simulink model "wavelet_transform_int"  (R2024b)
settings: Solver=FixedStepDiscrete  StartTime=0.0  StopTime=10.0  RelTol=1e-3
InitFcn:
  | n=50;
  | 
  | fprintf('Size of matrix A: n = %d\n', n);
libraries: simulink x1
settings Model: DataTypeOverride=Off  Creator=valen  LastModifiedBy=valen
settings SolverCC: AlgebraicLoopSolver=TrustRegion
settings DataIOCC: LimitDataPoints=on  SaveOutput=off  SaveTime=off
settings OptimizationCC: BlockReduction=off  ConditionallyExecuteInputs=off  DefaultParameterBehavior=Inlined  LifeSpan=inf
settings DebuggingCC: AlgebraicLoopMsg=error  SingleTaskRateTransMsg=error  UnconnectedInputMsg=warning  UnconnectedOutputMsg=warning  UnconnectedLineMsg=warning  AllowSymbolicDim=off  StrictBusMsg=ErrorOnBusTreatedAsVector  SFUnexpectedBacktrackingDiag=warning  SFNoUnconditionalDefaultTransitionDiag=warning  SFExecutionAtInitializationDiag=none  ArithmeticOperatorsInVariantConditions=warning
settings HardwareCC: ProdBitPerPointer=32  ProdBitPerSizeT=32  ProdBitPerPtrDiffT=32  ProdLargestAtomicFloat=None  ProdIntDivRoundTo=Undefined  ProdEndianess=Unspecified  ProdWordSize=32  ProdHWDeviceType=ASIC/FPGA->ASIC/FPGA  ProdEqTarget=off
settings ModelReferenceCC: EnableRefExpFcnMdlSchedulingChecks=on
settings SFSimCC: SimUseLocalCustomCode=off  CustomCodeUndefinedFunction=UseInterfaceOnly
settings RTWCC: RTWUseLocalCustomCode=off  GPUComputeCapability=3.5
settings CodeAppCC: StateflowObjectComments=on
settings GRTTargetCC: TargetLangStandard=C89/C90 (ANSI)
settings ConfigComp: CovScope=ReferencedModels  CovMetricSettings=dw  CovSaveCumulativeToWorkspaceVar=on  CovSaveSingleToWorkspaceVar=on  CovExternalEMLEnable=off  CovSFcnEnable=off

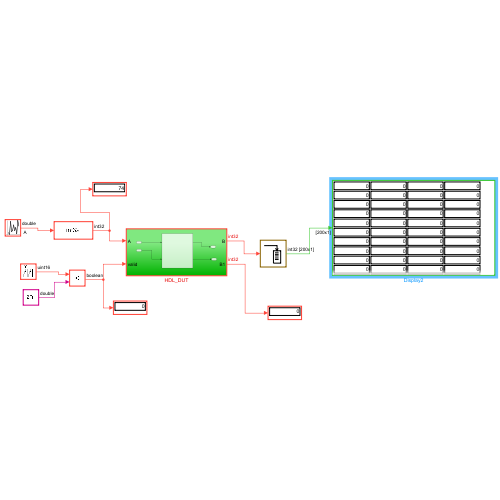
[thumbnail: Simulink's stored preview of the top-level diagram]
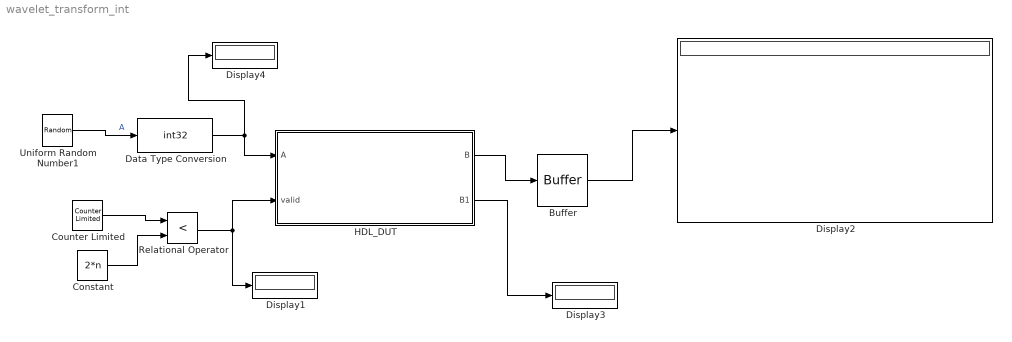
== system wavelet_transform_int ==
  Buffer : Buffer  N=4*n  OutputFrames=off
  Constant : Constant  Value=2*n
  Counter Limited : simulink/Sources/Counter Limited  uplimit=n*(n+1)  tsamp=-1
  Data Type Conversion : DataTypeConversion  OutDataTypeStr=int32  SaturateOnIntegerOverflow=off  RndMeth=Floor
  Display{1..4} (4 alike) : Display
  HDL_DUT : Subsystem
  Relational Operator : RelationalOperator  Operator=<  OutDataTypeStr=boolean  RndMeth=Simplest  InputSameDT=off
  Uniform Random Number1 : UniformRandomNumber  Minimum=0  Maximum=100  Seed=n  SampleTime=10/(4*n+1)
  wires:
  Data Type Conversion/1 -> HDL_DUT/1(A), Display4/1
  Relational Operator/1 -> HDL_DUT/2(valid), Display1/1
  Counter Limited/1 -> Relational Operator/1
  Constant/1 -> Relational Operator/2
  Buffer/1 -> Display2/1
  HDL_DUT/1(B) -> Buffer/1
  Uniform Random Number1/1 -> Data Type Conversion/1  "A"
  HDL_DUT/2(B1) -> Display3/1

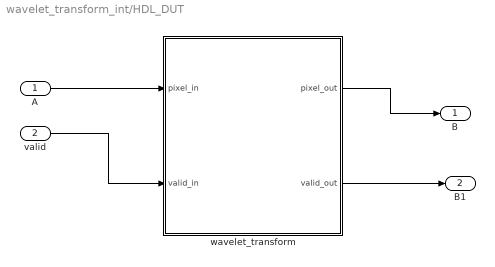
== system wavelet_transform_int/HDL_DUT ==
  A : Inport
  valid : Inport  Port=2
  wavelet_transform : MATLAB Function  TreatAsAtomicUnit=on
  B : Outport  VectorParamsAs1DForOutWhenUnconnected=off
  B1 : Outport  Port=2  VectorParamsAs1DForOutWhenUnconnected=off
  wires:
  A/1 -> wavelet_transform/1(pixel_in)
  valid/1 -> wavelet_transform/2(valid_in)
  wavelet_transform/1(pixel_out) -> B/1
  wavelet_transform/2(valid_out) -> B1/1

== matlab function wavelet_transform_int/HDL_DUT/wavelet_transform ==
  data: pixel_in input; pixel_out output; valid_in input; valid_out output
function [pixel_out,valid_out] = hardware_walevet_transform(pixel_in, valid_in)
    WIDTH = 50;
    TOTAL_PIXELS =2*WIDTH;
    
    % Registres persistants (Hardware)
    persistent bufferA bufferB count state;
    if isempty(state)
        bufferA = zeros(1, TOTAL_PIXELS, 'int32');% RAM de stockage temporaire
        bufferB=zeros(1, WIDTH, 'int32');
        count = int32(1);
        state = int32(0); % 0: Accumulation, 1: Calcul Inverse, 2: Stream Sortie
    end
    
    % Signaux de contrôle par défaut
    pixel_out = int32(0);
    valid_out = int32(0);
    
    switch state
        case 0 % --- PASSE 1 : ACCUMULATION & STOCKAGE ---
            if valid_in
                 % 2. Stockage dans la mémoire tampon
                bufferA(count) = int32(pixel_in);
                
                if count == TOTAL_PIXELS
                    count = int32(0);
                    state = int32(1); % Matrice reçue -> Passe à l'étape suivante
                else
                    count = count + 1;
                end               
            end
            
        case 1 % --- high_part ---
            if count == 0
			   sum_value_high = bufferA(2) - int32((0.5625 * (bufferA(1) + bufferA(3))) - (0.0625 * (bufferA(3) + bufferA(5))) + 0.5);
            elseif count == WIDTH -2
			   sum_value_high = bufferA(2*WIDTH - 2) - int32((0.5625 * (bufferA(2*WIDTH -3) + bufferA(2*WIDTH -1))) - (0.0625 * (bufferA(2*WIDTH - 5) + bufferA(2*WIDTH - 1))) + 0.5);
            elseif count == WIDTH - 1
			   sum_value_high = bufferA(2*WIDTH) - int32( (1.125 * (bufferA(2*WIDTH -1))) -  (0.125 * (bufferA(2*WIDTH - 3))) + 0.5);
            else
			   % generic case
			   sum_value_high = bufferA(2*count+2) - int32( ((0.5625) * (bufferA(2*count+1) + bufferA(2*count+3))) - (0.0625 * (bufferA(2*count - 1) + bufferA(2*count + 5))) + 0.5);
            end
            
            pixel_out=sum_value_high;
            bufferB(count+1)=sum_value_high;

            if count ==WIDTH-1
                % Réinitialisation pour la matrice suivante
                count = int32(0);
                state = int32(2); 
                valid_out = int32(1); % End of highpart calculation
            else
                count = count + 1;
            end

        case 2 % --- low_part ---
            if count == 0
			    pixel_out = bufferA(1) - int32(- (bufferB(1)*0.5) + 0.5);
            else
			    pixel_out = bufferA(2*count+1) - int32( - (( bufferB(count) +  bufferB(count+1))*0.25) + 0.5);
            end
		                    
            if count ==WIDTH-1
                % Réinitialisation pour la matrice suivante
                count = int32(1);
                state = int32(0); 
                valid_out = int32(2);% End of low_part calculation  
            else
                count = count + 1;
            end
    end
end
